simulink model "ControlLoopCont"  (R2024a)
settings: Solver=VariableStepAuto  StartTime=0.0  StopTime=10.0  RelTol=1e-3
values from neighbouring files (symbols this model uses):
  g = 9.80665    [VariableLoader.m]
  l = 3.7    [VariableLoader.m]
undefined symbols (not defined in the file or in its folder): C
settings Model: Creator=Riley  LastModifiedBy=Riley

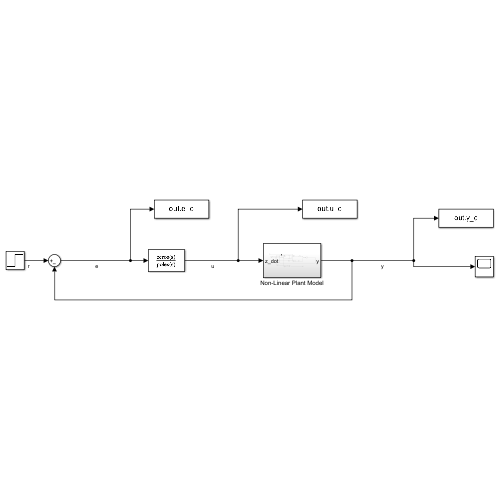
[thumbnail: Simulink's stored preview of the top-level diagram]
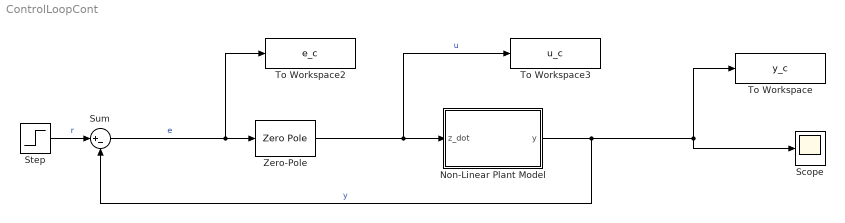
== system ControlLoopCont ==
  Non-Linear Plant Model : Subsystem
  Scope : Scope
  Step : Step  Time=0  SampleTime=0
  Sum : Sum  Inputs=|+-
  To Workspace : ToWorkspace  VariableName=y_c  SaveFormat=Timeseries  SampleTime=-1
  To Workspace2 : ToWorkspace  VariableName=e_c  SaveFormat=Timeseries  SampleTime=-1
  To Workspace3 : ToWorkspace  VariableName=u_c  SaveFormat=Timeseries  SampleTime=-1
  Zero-Pole : ZeroPole  Zeros=C.Z{1}  Poles=C.P{1}  Gain=C.K
  wires:
  Non-Linear Plant Model/1(y) -> Sum/2, To Workspace/1, Scope/1  "y"
  Zero-Pole/1 -> To Workspace3/1, Non-Linear Plant Model/1(z_dot)  "u"
  Step/1 -> Sum/1  "r"
  Sum/1 -> Zero-Pole/1, To Workspace2/1  "e"

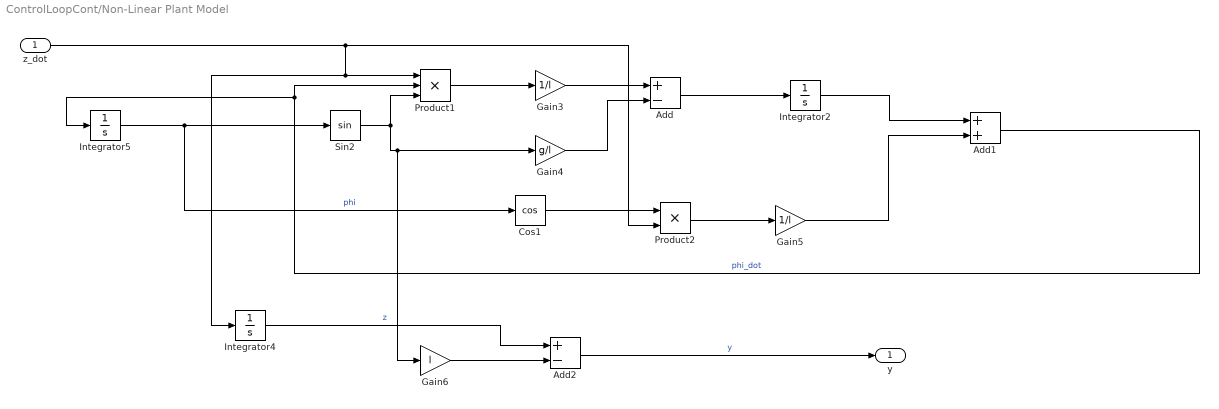
== system ControlLoopCont/Non-Linear Plant Model ==
  z_dot : Inport
  Add : Sum  Inputs=+-
  Add1 : Sum
  Add2 : Sum  Inputs=+-
  Cos1 : Trigonometry  Operator=cos
  Gain3 : Gain  Gain=1/l
  Gain4 : Gain  Gain=g/l
  Gain5 : Gain  Gain=1/l
  Gain6 : Gain  Gain=l
  Integrator2 : Integrator
  Integrator4 : Integrator
  Integrator5 : Integrator
  Product1 : Product  Inputs=3
  Product2 : Product
  Sin2 : Trigonometry
  y : Outport
  wires:
  z_dot/1 -> Integrator4/1, Product1/1, Product2/2
  Sin2/1 -> Gain4/1, Gain6/1, Product1/3
  Product1/1 -> Gain3/1
  Add1/1 -> Product1/2, Integrator5/1  "phi_dot"
  Gain3/1 -> Add/1
  Integrator5/1 -> Cos1/1, Sin2/1  "phi"
  Integrator2/1 -> Add1/1
  Add/1 -> Integrator2/1
  Cos1/1 -> Product2/1
  Product2/1 -> Gain5/1
  Gain4/1 -> Add/2
  Gain5/1 -> Add1/2
  Gain6/1 -> Add2/2
  Integrator4/1 -> Add2/1  "z"
  Add2/1 -> y/1  "y"
